simulink model "New_Grashof"  (Simulink 7.9)
settings: Solver=FixedStepDiscrete  StartTime=0.0  StopTime=10  FixedStep=1  RelTol=1e-3
undefined symbols (not defined in the file): Carnot_Grashof_Callbacks
settings Model: Creator=awohlfei  LastModifiedBy=awohlfei

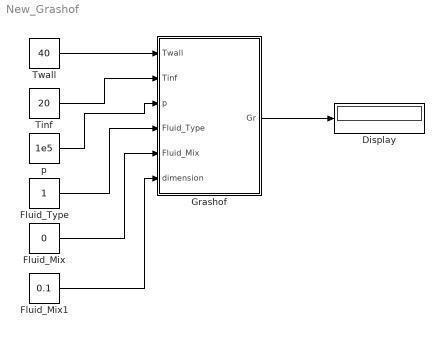
== system New_Grashof ==
  Display : Display
  Fluid_Mix : Constant  Value=0
  Fluid_Mix1 : Constant  Value=0.1
  Fluid_Type : Constant
  Grashof : Subsystem  LoadFcn=Carnot_Grashof_Callbacks('LoadFcn');  VariantObject=CarlibClassic  mask(Grashof){DEBUGLEVEL=WARNING, MAXTOTALMESSAGES=inf, MAXCONSECUTIVEMESSAGES=inf, WRITETOFILE=0, FILENAME='errors.txt'}
      mask prompts: DEBUGLEVEL "Debug level"; MAXTOTALMESSAGES "maximum number of total warning"; MAXCONSECUTIVEMESSAGES "maximum number of consecutive warnings"; WRITETOFILE "write messages to file"; FILENAME "filename for error messages"
      mask help:
      | Calculates the Gashof number. Inputs are:
      | 1   wall temperature
      | 2   temperature at infinite distance
      | 3   pressure
      | 4   fluid type (see below)
      | 5   fluid_mix
      | 6   characteristic dimension
      |
      | Definition of the fluid types
      |  1        water
      |  2        air                    fluid_mix is (kg water) / (kg air)
      |  3        cotton oil
      |  4        silicone oil
      |  5        water-glycol    fluid_mix gives the volume-percent of glycol
      |  6        tyfocor LS      only available in liquid phase
      mask init:
      | %global debug level
      | [DEBUGLEVEL, MAXTOTALMESSAGES, MAXCONSECUTIVEMESSAGES, WRITETOFILE, FILENAME] = Carnot_Grashof_Callbacks('CheckDebugLevels', DEBUGLEVEL, MAXTOTALMESSAGES, MAXCONSECUTIVEMESSAGES, WRITETOFILE, FILENAME);
      mask Help: eval('man(''grashof'')')
      mask StyleString: popup(DEBUG|INFO|WARNING|ERROR|FATAL|NONE),edit,edit,edit,edit
      mask TabNameString: Debugging,Debugging,Debugging,Debugging,Debugging
  Tinf : Constant  Value=20
  Twall : Constant  Value=40
  p : Constant  Value=1e5
  wires:
  Twall/1 -> Grashof/1(Twall)
  p/1 -> Grashof/3(p)
  Fluid_Type/1 -> Grashof/4(Fluid_Type)
  Fluid_Mix/1 -> Grashof/5(Fluid_Mix)
  Grashof/1(Gr) -> Display/1
  Fluid_Mix1/1 -> Grashof/6(dimension)
  Tinf/1 -> Grashof/2(Tinf)

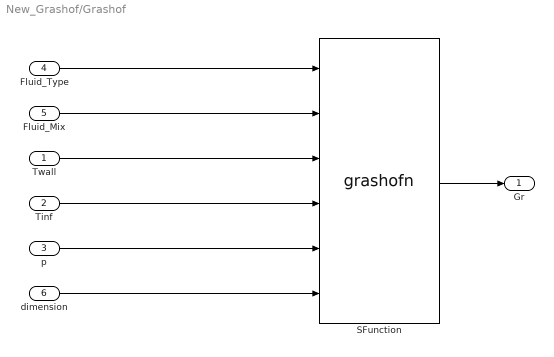
== system New_Grashof/Grashof ==
  Twall : Inport
  Tinf : Inport  Port=2
  p : Inport  Port=3
  Fluid_Type : Inport  Port=4
  Fluid_Mix : Inport  Port=5
  dimension : Inport  Port=6
  SFunction : S-Function  FunctionName=grashofn  Parameters=DEBUGLEVEL,MAXTOTALMESSAGES,MAXCONSECUTIVEMESSAGES,WRITETOFILE,FILENAME  EnableBusSupport=off
  Gr : Outport
  wires:
  SFunction/1 -> Gr/1
  Fluid_Type/1 -> SFunction/1
  Fluid_Mix/1 -> SFunction/2
  Twall/1 -> SFunction/3
  Tinf/1 -> SFunction/4
  p/1 -> SFunction/5
  dimension/1 -> SFunction/6
